simulink model "OcularMotorLabModel_2023_08_25_M23a"  (R2023a)
settings: Solver=FixedStepAuto  StartTime=tStart  StopTime=tFinal  FixedStep=0.001  RelTol=1e-3
undefined symbols (not defined in the file or in its folder): Asp, Asp1, Asp2, e0sp, gaussian, Gpc, GPos, Gsl, psi, Psp1, RotFbk, SacThDeg, SatSp, sigbuilder_block, SomFbk, T1, T2, Tccanal, Tcn, Tcr, Tcsp, TCvs, tdm, tdsp1, tdsp2, tdsp3, tdv, Tsl, Tz, w
libraries: matrix_library x10, vrlib x9, simulink_extras x5, simulink x2
(part 2 of 2)

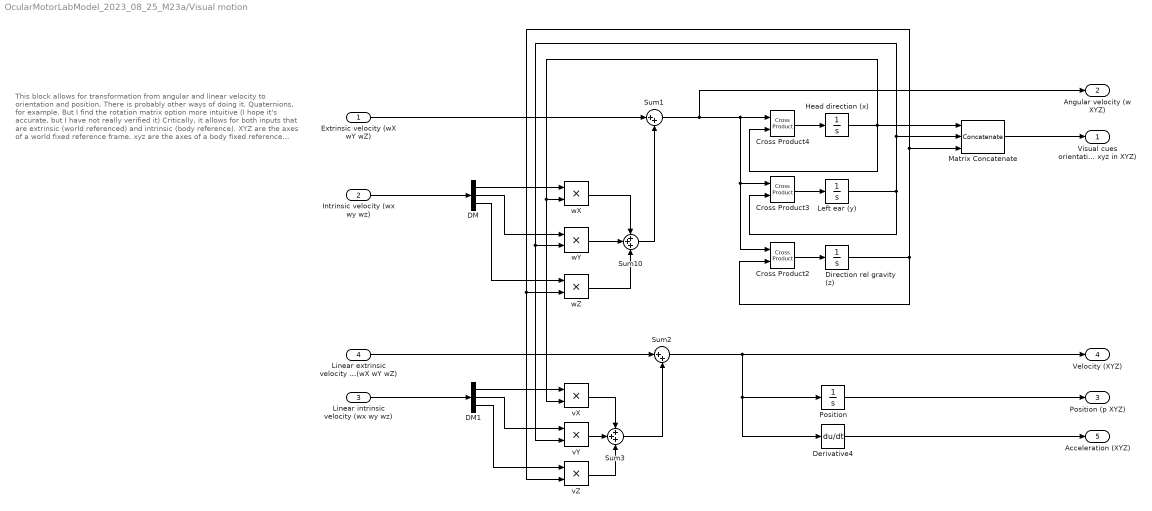
== system OcularMotorLabModel_2023_08_25_M23a/Visual motion ==
  note: This block allows for transformation from angular and linear velocity to orientation and position. There is probably other ways of doing it. Quaternions, for example. But I find the rotation matrix option more intuitive (I hope it's accurate, but I have not really verified it)
      |
      | Critically, it allows for both inputs that are extrinsic (world referenced) and intrinsic (body reference).
      |
      | XYZ are the axes of a world fixed reference frame.
      | xyz are the axes of a body fixed reference frame
      |
      | For the extrinsic angular velocities, they need to be integrated after a cross product with each of the xyz axis, that way they provide the rotation of such axis within the XYZ world fixed reference frame.
      |
      | For the intrinsic angular velocities, they simply multiply each of the intrisic axis and get added to the extrinsic velocities.
      |
      | A similar approach is followed for the linear velocities but without the cross products are linear velocities can be simply integrated by components.
  Extrinsic velocity (wX wY wZ) : Inport
  Intrinsic velocity (wx wy wz) : Inport  Port=2
  Linear intrinsic velocity (wx wy wz) : Inport  Port=3
  Linear extrinsic velocity (wX wY wZ) : Inport  Port=4
  Cross Product2 : vrlib/Utilities/Cross Product
  Cross Product3 : vrlib/Utilities/Cross Product
  Cross Product4 : vrlib/Utilities/Cross Product
  DM : Demux  Outputs=3
  DM1 : Demux  Outputs=3
  Derivative4 : Derivative
  Direction rel gravity (z) : Integrator  InitialCondition=[0 0 1]
  Head direction (x) : Integrator  InitialCondition=[1 0 0]
  Left ear (y) : Integrator  InitialCondition=[0 1 0]
  Matrix Concatenate : Concatenate  NumInputs=3  Mode=Multidimensional array  ConcatenateDimension=2
  Position : Integrator  InitialCondition=[0 0 0]
  Sum1 : Sum  Inputs=|++
  Sum10 : Sum  Inputs=+++
  Sum2 : Sum  Inputs=|++
  Sum3 : Sum  Inputs=+++
  vX : Product
  vY : Product
  vZ : Product
  wX : Product
  wY : Product
  wZ : Product
  Visual cues orientation in world (R xyz in XYZ) : Outport
  Angular velocity (w XYZ) : Outport  Port=2
  Position (p XYZ) : Outport  Port=3
  Velocity (XYZ) : Outport  Port=4
  Acceleration (XYZ) : Outport  Port=5
  wires:
  Head direction (x)/1 -> Cross Product4/2, wX/2, vX/2, Matrix Concatenate/1
  Cross Product4/1 -> Head direction (x)/1
  Direction rel gravity (z)/1 -> Matrix Concatenate/3, wZ/2, vZ/2, Cross Product2/2
  Cross Product2/1 -> Direction rel gravity (z)/1
  Left ear (y)/1 -> Matrix Concatenate/2, vY/2, wY/2, Cross Product3/2
  Sum1/1 -> Cross Product2/1, Cross Product3/1, Cross Product4/1, Angular velocity (w XYZ)/1
  Cross Product3/1 -> Left ear (y)/1
  DM/1 -> wX/1
  DM/2 -> wY/1
  DM/3 -> wZ/1
  wX/1 -> Sum10/1
  wY/1 -> Sum10/2
  wZ/1 -> Sum10/3
  Sum10/1 -> Sum1/2
  Position/1 -> Position (p XYZ)/1
  vY/1 -> Sum3/2
  DM1/2 -> vY/1
  vZ/1 -> Sum3/3
  DM1/3 -> vZ/1
  DM1/1 -> vX/1
  vX/1 -> Sum3/1
  Sum3/1 -> Sum2/2
  Matrix Concatenate/1 -> Visual cues orientation in world (R xyz in XYZ)/1
  Sum2/1 -> Position/1, Derivative4/1, Velocity (XYZ)/1
  Derivative4/1 -> Acceleration (XYZ)/1
  Intrinsic velocity (wx wy wz)/1 -> DM/1
  Linear extrinsic velocity (wX wY wZ)/1 -> Sum2/1
  Linear intrinsic velocity (wx wy wz)/1 -> DM1/1
  Extrinsic velocity (wX wY wZ)/1 -> Sum1/1

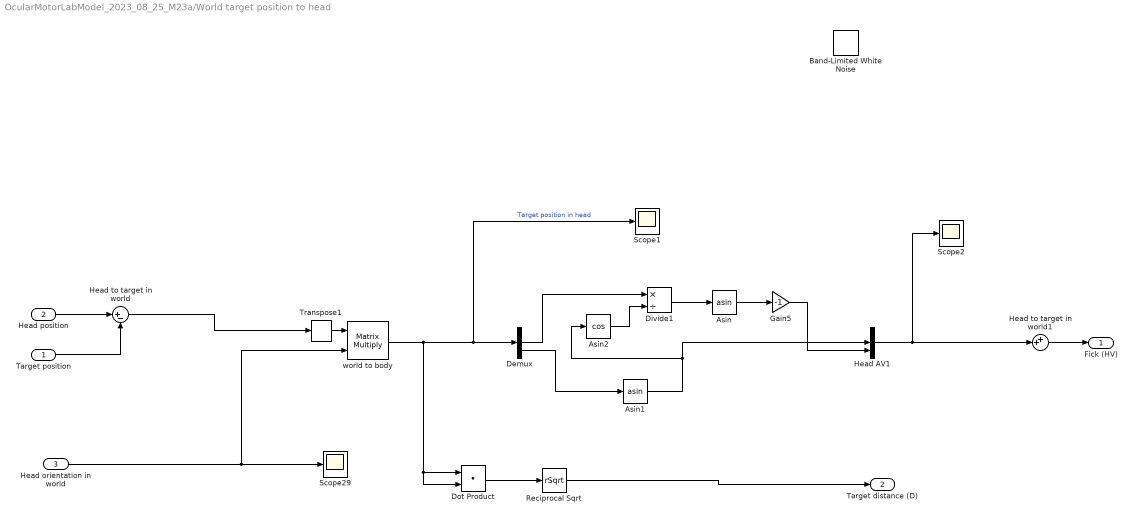
== system OcularMotorLabModel_2023_08_25_M23a/World target position to head ==
  Target position : Inport
  Head position : Inport  Port=2
  Head orientation in world : Inport  Port=3
  Asin : Trigonometry  Operator=asin
  Asin1 : Trigonometry  Operator=asin
  Asin2 : Trigonometry  Operator=cos
  Band-Limited White Noise : simulink/Sources/Band-Limited White Noise  Cov=[0.00000000001]  Ts=0.002  seed=[23341]
  Demux : Demux  Outputs=3
  Divide1 : Product  Inputs=*/
  Dot Product : DotProduct  OutDataTypeStr=Inherit: Inherit via internal rule
  Gain5 : Gain  Gain=-1
  Head AV1 : Mux  Inputs=3
  Head to target in world : Sum  Inputs=|+-
  Head to target in world1 : Sum  Inputs=++|
  Reciprocal Sqrt : Sqrt  Operator=rSqrt
  Scope1 : Scope
  Scope2 : Scope
  Scope29 : Scope
  Transpose1 : matrix_library/Transpose
  world to body : Product  Multiplication=Matrix(*)
  Fick (HV) : Outport
  Target distance (D) : Outport  Port=2
  wires:
  world to body/1 -> Dot Product/2, Dot Product/1, Scope1/1, Demux/1  "Target position in head"
  Target position/1 -> Head to target in world/2
  Head position/1 -> Head to target in world/1
  Head to target in world/1 -> Transpose1/1
  Head orientation in world/1 -> world to body/2, Scope29/1
  Asin/1 -> Gain5/1
  Demux/3 -> Asin1/1
  Asin1/1 -> Asin2/1, Head AV1/2
  Head AV1/1 -> Scope2/1, Head to target in world1/2
  Transpose1/1 -> world to body/1
  Demux/2 -> Divide1/1
  Asin2/1 -> Divide1/2
  Divide1/1 -> Asin/1
  Gain5/1 -> Head AV1/3
  Dot Product/1 -> Reciprocal Sqrt/1
  Reciprocal Sqrt/1 -> Target distance (D)/1
  Head to target in world1/1 -> Fick (HV)/1

== system OcularMotorLabModel_2023_08_25_M23a/World to canals ==
  Head orientation : Inport
  Head velocity : Inport  Port=2
  Canal orientations1 : Constant  Value=[1 0 0;0 1 0;0 0 1]  VectorParams1D=off
  Transpose : matrix_library/Transpose
  Transpose1 : matrix_library/Transpose
  world to body : Product  Multiplication=Matrix(*)
  world to body1 : Product  Multiplication=Matrix(*)
  Out1 : Outport
  wires:
  Transpose/1 -> Out1/1
  world to body1/1 -> Transpose/1  "Head velocity"
  Head orientation/1 -> world to body/2
  world to body/1 -> world to body1/1  "Head velocity"
  Head velocity/1 -> Transpose1/1
  Transpose1/1 -> world to body/1
  Canal orientations1/1 -> world to body1/2

== system OcularMotorLabModel_2023_08_25_M23a/World to head ==
  note: GIa is calculated as the vector sum of G and linear acceleration in body reference
  Orientation : Inport
  Linear acceleration : Inport  Port=2
  1/G : Gain  Gain=1/9.8
  G (XYZ) : Constant  Value=[0 0 -1]  VectorParams1D=off
  Rotate gravity to body coordinates : Product  Multiplication=Matrix(*)
  Rotate gravity to body coordinates1 : Product  Multiplication=Matrix(*)
  Sum : Sum  Inputs=++|
  Transpose : matrix_library/Transpose
  Transpose1 : matrix_library/Transpose
  Transpose2 : matrix_library/Transpose
  GIA (in Gs) : Outport
  wires:
  Linear acceleration/1 -> Transpose/1
  Orientation/1 -> Rotate gravity to body coordinates/2, Rotate gravity to body coordinates1/2
  Rotate gravity to body coordinates/1 -> Transpose1/1
  G (XYZ)/1 -> Rotate gravity to body coordinates/1
  Sum/1 -> GIA (in Gs)/1  "GIA"
  1/G/1 -> Rotate gravity to body coordinates1/1
  Rotate gravity to body coordinates1/1 -> Transpose2/1
  Transpose/1 -> 1/G/1
  Transpose1/1 -> Sum/1
  Transpose2/1 -> Sum/2

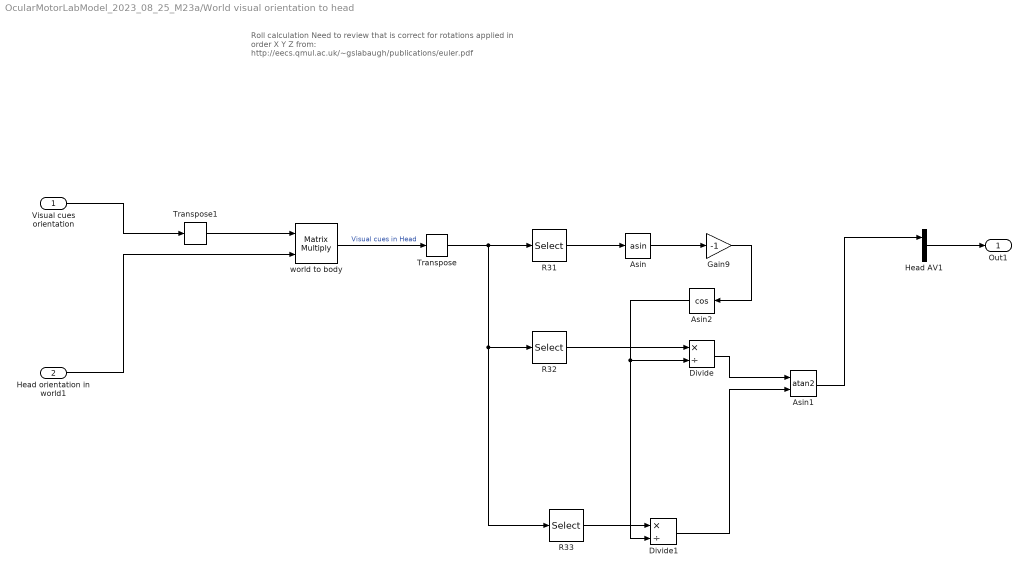
== system OcularMotorLabModel_2023_08_25_M23a/World visual orientation to head ==
  note: Roll calculation
      |
      | Need to review that is correct for rotations applied in order X Y Z
      |
      | from: http://eecs.qmul.ac.uk/~gslabaugh/publications/euler.pdf
  Visual cues orientation : Inport
  Head orientation in world1 : Inport  Port=2
  Asin : Trigonometry  Operator=asin
  Asin1 : Trigonometry  Operator=atan2
  Asin2 : Trigonometry  Operator=cos
  Divide : Product  Inputs=*/
  Divide1 : Product  Inputs=*/
  Gain9 : Gain  Gain=-1
  Head AV1 : Mux  Inputs=3
  R31 : Selector  NumberOfDimensions=2  InputPortWidth=3  IndexOptions=Index vector (dialog),Index vector (dialog)  Indices=3,1  OutputSizes=1,1
  R32 : Selector  NumberOfDimensions=2  InputPortWidth=3  IndexOptions=Index vector (dialog),Index vector (dialog)  Indices=3,2  OutputSizes=1,1
  R33 : Selector  NumberOfDimensions=2  InputPortWidth=3  IndexOptions=Index vector (dialog),Index vector (dialog)  Indices=3,3  OutputSizes=1,1
  Transpose : matrix_library/Transpose
  Transpose1 : matrix_library/Transpose
  world to body : Product  Multiplication=Matrix(*)
  Out1 : Outport
  wires:
  Transpose/1 -> R31/1, R32/1, R33/1
  world to body/1 -> Transpose/1  "Visual cues in Head"
  Visual cues orientation/1 -> Transpose1/1
  Head orientation in world1/1 -> world to body/2
  Gain9/1 -> Asin2/1
  Asin1/1 -> Head AV1/1
  Head AV1/1 -> Out1/1
  R31/1 -> Asin/1
  R32/1 -> Divide/1
  Asin/1 -> Gain9/1
  R33/1 -> Divide1/1
  Divide1/1 -> Asin1/2
  Divide/1 -> Asin1/1
  Transpose1/1 -> world to body/1
  Asin2/1 -> Divide1/2, Divide/2

== system OcularMotorLabModel_2023_08_25_M23a/World visual velocity  to head ==
  Visual velocity in world : Inport
  Head orientation in world : Inport  Port=2
  Transpose : matrix_library/Transpose
  Transpose1 : matrix_library/Transpose
  world to body : Product  Multiplication=Matrix(*)
  Out1 : Outport
  wires:
  Head orientation in world/1 -> world to body/2
  Visual velocity in world/1 -> Transpose1/1
  world to body/1 -> Transpose/1  "Visual velocity in Head"
  Transpose1/1 -> world to body/1
  Transpose/1 -> Out1/1

== system OcularMotorLabModel_2023_08_25_M23a/Head velocity (body)/Subsystem ==
  In1 : Inport
  Demux : Demux  Tag=STV Demux  Outputs=3
      settings: DisplayOption=none
  nasooccipital : Outport  Tag=STV Outport
  interaural : Outport  Tag=STV Outport  Port=2
  rostrocaudal : Outport  Tag=STV Outport  Port=3
  wires:
  Demux/1 -> nasooccipital/1
  Demux/2 -> interaural/1
  Demux/3 -> rostrocaudal/1
  In1/1 -> Demux/1

== system OcularMotorLabModel_2023_08_25_M23a/Head velocity (world)/Subsystem ==
  In1 : Inport
  Demux : Demux  Tag=STV Demux  Outputs=3
      settings: DisplayOption=none
  x : Outport  Tag=STV Outport
  y : Outport  Tag=STV Outport  Port=2
  z : Outport  Tag=STV Outport  Port=3
  wires:
  Demux/1 -> x/1
  Demux/2 -> y/1
  Demux/3 -> z/1
  In1/1 -> Demux/1

== system OcularMotorLabModel_2023_08_25_M23a/Linear body velocity/Subsystem ==
  Demux : Demux  Tag=STV Demux  Outputs=3
      settings: DisplayOption=none

== system OcularMotorLabModel_2023_08_25_M23a/Linear world velocity/Subsystem ==
  Demux : Demux  Tag=STV Demux  Outputs=3
      settings: DisplayOption=none

== system OcularMotorLabModel_2023_08_25_M23a/Only for simulations of spv/Left eye plant1 ==
  In1 : Inport
  Demux : Demux  Outputs=3
  Mux : Mux  Inputs=3
  Plant1 : TransferFcn  Numerator=[Tz 1]  Denominator=[T1*T2 (T1+T2) 1]
  Plant2 : TransferFcn  Numerator=[w^2]  Denominator=[1 + 2*psi*w w^2]
  Plant3 : TransferFcn  Numerator=[Tz 1]  Denominator=[T1*T2 (T1+T2) 1]
  Plant4 : TransferFcn  Numerator=[w^2]  Denominator=[1 + 2*psi*w w^2]
  Plant5 : TransferFcn  Numerator=[Tz 1]  Denominator=[T1*T2 (T1+T2) 1]
  Plant6 : TransferFcn  Numerator=[w^2]  Denominator=[1 + 2*psi*w w^2]
  Saturation : Saturate  UpperLimit=50*pi/180  LowerLimit=-50*pi/180
  Eye position : Outport
  wires:
  In1/1 -> Demux/1
  Mux/1 -> Saturation/1  "Eye position"
  Plant4/1 -> Mux/1
  Plant2/1 -> Mux/2
  Plant6/1 -> Mux/3
  Demux/1 -> Plant3/1
  Demux/2 -> Plant1/1
  Demux/3 -> Plant5/1
  Saturation/1 -> Eye position/1
  Plant3/1 -> Plant4/1
  Plant1/1 -> Plant2/1
  Plant5/1 -> Plant6/1

== system OcularMotorLabModel_2023_08_25_M23a/Pursuit  corollary/Eye plant ==
  In1 : Inport
  Demux : Demux  Outputs=3
  Mux : Mux  Inputs=3
  Plant1 : TransferFcn  Numerator=[Tz 1]  Denominator=[T1*T2 (T1+T2) 1]
  Plant2 : TransferFcn  Numerator=[w^2]  Denominator=[1 + 2*psi*w w^2]
  Plant3 : TransferFcn  Numerator=[Tz 1]  Denominator=[T1*T2 (T1+T2) 1]
  Plant4 : TransferFcn  Numerator=[w^2]  Denominator=[1 + 2*psi*w w^2]
  Plant5 : TransferFcn  Numerator=[Tz 1]  Denominator=[T1*T2 (T1+T2) 1]
  Plant6 : TransferFcn  Numerator=[w^2]  Denominator=[1 + 2*psi*w w^2]
  Eye position : Outport
  wires:
  In1/1 -> Demux/1
  Mux/1 -> Eye position/1  "Eye position"
  Plant4/1 -> Mux/1
  Plant2/1 -> Mux/2
  Plant6/1 -> Mux/3
  Demux/1 -> Plant3/1
  Demux/2 -> Plant1/1
  Demux/3 -> Plant5/1
  Plant3/1 -> Plant4/1
  Plant1/1 -> Plant2/1
  Plant5/1 -> Plant6/1

== system OcularMotorLabModel_2023_08_25_M23a/Saccade corollary/Eye plant ==
  In1 : Inport
  Demux : Demux  Outputs=3
  Mux : Mux  Inputs=3
  Plant1 : TransferFcn  Numerator=[Tz 1]  Denominator=[T1*T2 (T1+T2) 1]
  Plant2 : TransferFcn  Numerator=[w^2]  Denominator=[1 + 2*psi*w w^2]
  Plant3 : TransferFcn  Numerator=[Tz 1]  Denominator=[T1*T2 (T1+T2) 1]
  Plant4 : TransferFcn  Numerator=[w^2]  Denominator=[1 + 2*psi*w w^2]
  Plant5 : TransferFcn  Numerator=[Tz 1]  Denominator=[T1*T2 (T1+T2) 1]
  Plant6 : TransferFcn  Numerator=[w^2]  Denominator=[1 + 2*psi*w w^2]
  Eye position : Outport
  wires:
  In1/1 -> Demux/1
  Mux/1 -> Eye position/1  "Eye position"
  Plant4/1 -> Mux/1
  Plant2/1 -> Mux/2
  Plant6/1 -> Mux/3
  Demux/1 -> Plant3/1
  Demux/2 -> Plant1/1
  Demux/3 -> Plant5/1
  Plant3/1 -> Plant4/1
  Plant1/1 -> Plant2/1
  Plant5/1 -> Plant6/1

== system OcularMotorLabModel_2023_08_25_M23a/Smooth pursuit/Left eye plant ==
  In1 : Inport
  Demux : Demux  Outputs=3
  Mux : Mux  Inputs=3
  Plant1 : TransferFcn  Numerator=[Tz 1]  Denominator=[T1*T2 (T1+T2) 1]
  Plant2 : TransferFcn  Numerator=[w^2]  Denominator=[1 + 2*psi*w w^2]
  Plant3 : TransferFcn  Numerator=[Tz 1]  Denominator=[T1*T2 (T1+T2) 1]
  Plant4 : TransferFcn  Numerator=[w^2]  Denominator=[1 + 2*psi*w w^2]
  Plant5 : TransferFcn  Numerator=[Tz 1]  Denominator=[T1*T2 (T1+T2) 1]
  Plant6 : TransferFcn  Numerator=[w^2]  Denominator=[1 + 2*psi*w w^2]
  Eye position : Outport
  wires:
  In1/1 -> Demux/1
  Mux/1 -> Eye position/1  "Eye position"
  Plant4/1 -> Mux/1
  Plant2/1 -> Mux/2
  Plant6/1 -> Mux/3
  Demux/1 -> Plant3/1
  Demux/2 -> Plant1/1
  Demux/3 -> Plant5/1
  Plant3/1 -> Plant4/1
  Plant1/1 -> Plant2/1
  Plant5/1 -> Plant6/1

== system OcularMotorLabModel_2023_08_25_M23a/Target position/Subsystem ==
  In1 : Inport
  Demux : Demux  Tag=STV Demux  Outputs=3
      settings: DisplayOption=none
  tX (m) : Outport  Tag=STV Outport  VectorParamsAs1DForOutWhenUnconnected=off
  tY (m) : Outport  Tag=STV Outport  Port=2  VectorParamsAs1DForOutWhenUnconnected=off
  tZ (m) : Outport  Tag=STV Outport  Port=3  VectorParamsAs1DForOutWhenUnconnected=off
  wires:
  Demux/1 -> tX (m)/1
  Demux/2 -> tY (m)/1
  Demux/3 -> tZ (m)/1
  In1/1 -> Demux/1

== system OcularMotorLabModel_2023_08_25_M23a/Visual World Extrinsic Orientation (only for unidirectional reotations)/Subsystem ==
  In1 : Inport
  Demux : Demux  Tag=STV Demux  Outputs=3
      settings: DisplayOption=none
  N-O (roll) : Outport  Tag=STV Outport
  I-A (pitch) : Outport  Tag=STV Outport  Port=2
  R-C (yaw) : Outport  Tag=STV Outport  Port=3
  wires:
  Demux/1 -> N-O (roll)/1
  Demux/2 -> I-A (pitch)/1
  Demux/3 -> R-C (yaw)/1
  In1/1 -> Demux/1

== system OcularMotorLabModel_2023_08_25_M23a/Visual World Extrinsic velocity/Subsystem ==
  In1 : Inport
  Demux : Demux  Tag=STV Demux  Outputs=3
      settings: DisplayOption=none
  N-O (roll) : Outport  Tag=STV Outport
  I-A (pitch) : Outport  Tag=STV Outport  Port=2
  R-C (yaw) : Outport  Tag=STV Outport  Port=3
  wires:
  Demux/1 -> N-O (roll)/1
  Demux/2 -> I-A (pitch)/1
  Demux/3 -> R-C (yaw)/1
  In1/1 -> Demux/1
